simulink model "SISOclosednonlinear"  (R2017b)
settings: Solver=VariableStepAuto  StartTime=0.0  StopTime=15  RelTol=1e-3
settings Model: Creator=ladislav  LastModifiedBy=Milan

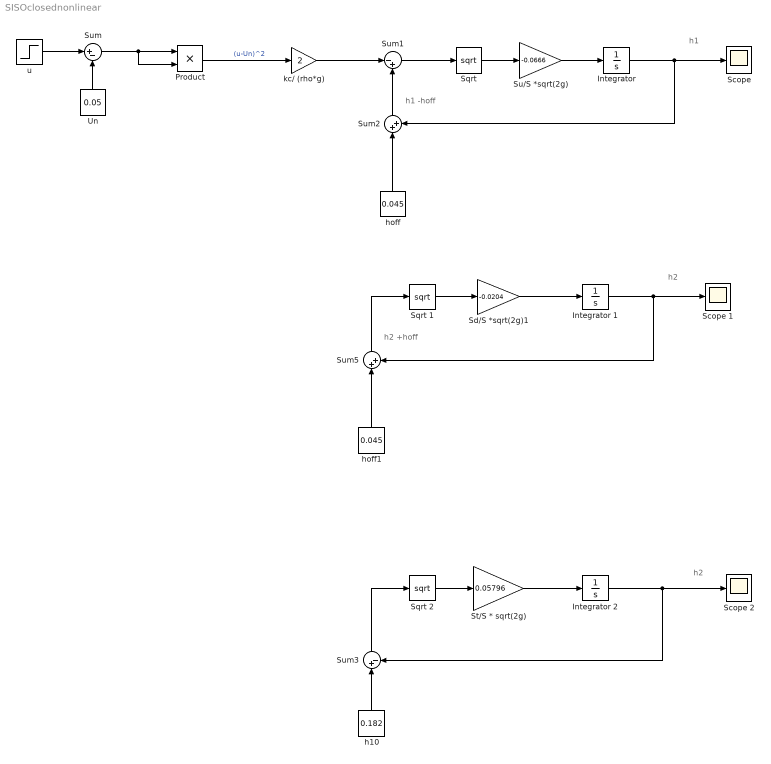
== system SISOclosednonlinear ==
  note: h1
  note: h1 -hoff
  note: h2 +hoff
  note: h2
  note: h2
  " Un" : Constant  Value=0.05
  " h10" : Constant  Value=0.182
  " hoff" : Constant  Value=0.045
  " hoff1" : Constant  Value=0.045
  "Integrator " : Integrator  InitialCondition=0.066
  Integrator 1 : Integrator  InitialCondition=0.175
  Integrator 2 : Integrator  InitialCondition=0.09
  "Product " : Product
  "Scope " : Scope
  Scope 1 : Scope
  Scope 2 : Scope
  Sd/S *sqrt(2g)1 : Gain  Gain=-0.0204
  "Sqrt " : Sqrt  SaturateOnIntegerOverflow=on
  Sqrt 1 : Sqrt  SaturateOnIntegerOverflow=on
  Sqrt 2 : Sqrt  SaturateOnIntegerOverflow=on
  "St/S * sqrt(2g) " : Gain  Gain=0.05796
  Su/S *sqrt(2g) : Gain  Gain=-0.0666
  Sum : Sum  Inputs=|+-
  Sum1 : Sum  Inputs=|-+
  Sum2 : Sum  Inputs=|++
  Sum3 : Sum  Inputs=|+-
  Sum5 : Sum  Inputs=|++
  kc/ (rho*g) : Gain  Gain=2
  u : Step  After=0  SampleTime=0
  wires:
  u/1 -> Sum/1
  " Un"/1 -> Sum/2
  Sum/1 -> "Product "/2, "Product "/1
  "Product "/1 -> kc/ (rho*g)/1  "(u-Un)^2"
  Sum1/1 -> "Sqrt "/1
  "Sqrt "/1 -> Su/S *sqrt(2g)/1
  Su/S *sqrt(2g)/1 -> "Integrator "/1
  Sum2/1 -> Sum1/2
  " hoff"/1 -> Sum2/1
  "Integrator "/1 -> "Scope "/1, Sum2/2
  " hoff1"/1 -> Sum5/1
  Sqrt 1/1 -> Sd/S *sqrt(2g)1/1
  Sd/S *sqrt(2g)1/1 -> Integrator 1/1
  Integrator 1/1 -> Scope 1/1, Sum5/2
  Sum5/1 -> Sqrt 1/1
  kc/ (rho*g)/1 -> Sum1/1
  Integrator 2/1 -> Sum3/2, Scope 2/1
  "St/S * sqrt(2g) "/1 -> Integrator 2/1
  Sqrt 2/1 -> "St/S * sqrt(2g) "/1
  Sum3/1 -> Sqrt 2/1
  " h10"/1 -> Sum3/1
